simulink model "Testing2"  (R2024b)
settings: Solver=FixedStepAuto  StartTime=0.0  StopTime=tspan  FixedStep=10  RelTol=1e-3
values from neighbouring files (symbols this model uses):
  E_b_ECI_0 = C2EulerAngles(C_b_ECI_0)    [FP_Solutions_Part_2_torque_free_init.m]    (also in test.m = quat2eul(q0))
  J = J.sc    [FP_Solutions_Part_2_torque_free_init.m]    (also in test.m = diag([1200,2000,2800]))
  q_b_ECI_0 = C2quat(C_b_ECI_0)    [FP_Solutions_Part_2_torque_free_init.m]    (also in test.m = [e0;n0])
  T = [0;0;0]    [FP_Solutions_Part_2_torque_free_init.m]    (also in test.m)
  w_b_ECI_0 = [0.001; -0.001; 0.002]    [FP_Solutions_Part_2_torque_free_init.m]    (also in test.m = [0.1; -0.05; 0.05])
settings Model: Creator=emehiel  LastModifiedBy=rosha
settings SolverCC: AlgebraicLoopSolver=TrustRegion
settings DebuggingCC: UnconnectedInputMsg=warning  UnconnectedOutputMsg=warning  UnconnectedLineMsg=warning
settings ModelReferenceCC: EnableRefExpFcnMdlSchedulingChecks=on
settings RTWCC: GPUComputeCapability=3.5

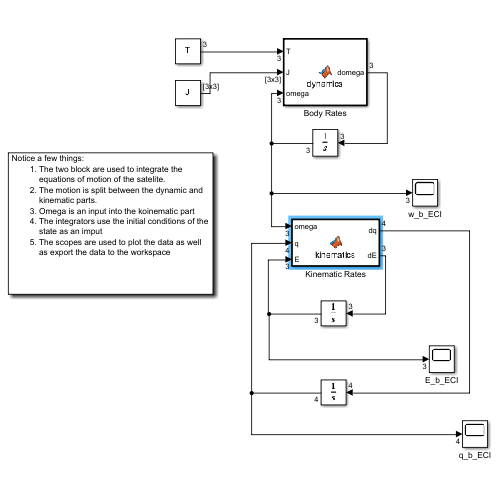
[thumbnail: Simulink's stored preview of the top-level diagram]
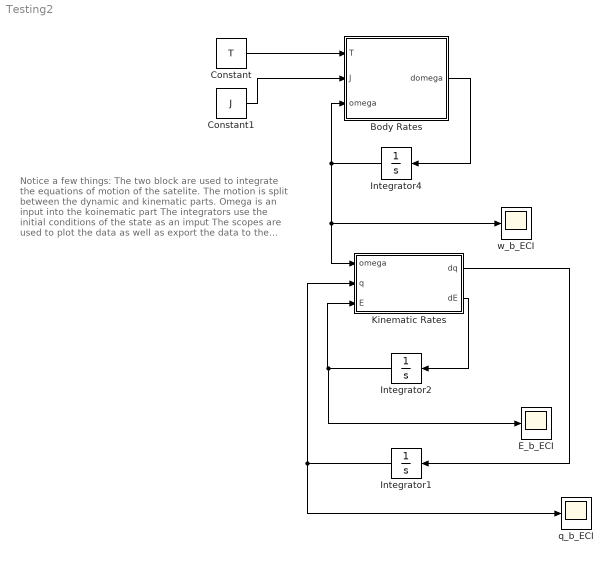
== system Testing2 ==
  note: Notice a few things:
      | The two block are used to integrate the equations of motion of the satelite.
      | The motion is split between the dynamic and kinematic parts.
      | Omega is an input into the koinematic part
      | The integrators use the initial conditions of the state as an imput
      | The scopes are used to plot the data as well as export the data to the workspace
  Body Rates : MATLAB Function  TreatAsAtomicUnit=on
  Constant : Constant  Value=T
  Constant1 : Constant  Value=J
  E_b_ECI : Scope
  Integrator1 : Integrator  InitialCondition=q_b_ECI_0
  Integrator2 : Integrator  InitialCondition=E_b_ECI_0
  Integrator4 : Integrator  InitialCondition=w_b_ECI_0
  Kinematic Rates : MATLAB Function  TreatAsAtomicUnit=on
  q_b_ECI : Scope
  w_b_ECI : Scope
  wires:
  Constant/1 -> Body Rates/1(T)
  Constant1/1 -> Body Rates/2(J)
  Body Rates/1(domega) -> Integrator4/1
  Integrator4/1 -> Body Rates/3(omega), w_b_ECI/1, Kinematic Rates/1(omega)
  Integrator2/1 -> E_b_ECI/1, Kinematic Rates/3(E)
  Integrator1/1 -> q_b_ECI/1, Kinematic Rates/2(q)
  Kinematic Rates/2(dE) -> Integrator2/1
  Kinematic Rates/1(dq) -> Integrator1/1

== matlab function Testing2/Kinematic Rates ==
  data: omega input; q input; dq output; E input; dE output
 function [dq,dE] = kinematics(omega, q, E)
%#codegen
% omega 3x1 
% q - 4x1 quaternion [q0; q1; q2; q3] 
% E - 3x1 Euler angles [roll; pitch; yaw] in radians
% Derivative of quaternion
wx = omega(1);
wy = omega(2);
wz = omega(3);
q0 = q(1);
q1 = q(2);
q2 = q(3);
q3 = q(4);
Omega = 0.5 * [ 0 -wx -wy -wz;
wx 0 wz -wy;
wy -wz 0 wx;
wz wy -wx 0 ];
dq = Omega * q;

phi = E(1); % roll
theta = E(2); % pitch
psi = E(3); % yaw

ph = E(1); % roll
th = E(2); % pitch
psi = E(3); % yaw

% Transformation matrix from Euler angle rates to omega
T = [1,      0,         -sin(theta);
     0, cos(phi),  cos(theta)*sin(phi);
     0, -sin(phi), cos(theta)*cos(phi)];

dE = T * omega;

== matlab function Testing2/Body Rates ==
  data: T input; J input; omega input; domega output
function domega = dynamics(T, J, omega)
    %#codegen
    % Compute the derivative of the angular velocity $\omega$ here
    
    domega = inv(J)*(T-vcross(omega)*J*omega);
    
    function [out] = vcross(v)
        out = [0, -v(3), v(2); v(3), 0, -v(1); -v(2), v(1), 0];
    end
end
